simulink model "Quadcopter Plant Feedback"  (R2023a)
settings: Solver=VariableStepAuto  StartTime=0.0  StopTime=10.0  RelTol=1e-3
undefined symbols (not defined in the file): Ax, Ay, b, d, g, Ixx, Izz, Jr, m
settings Model: Creator=NADJICH  LastModifiedBy=NADJICH

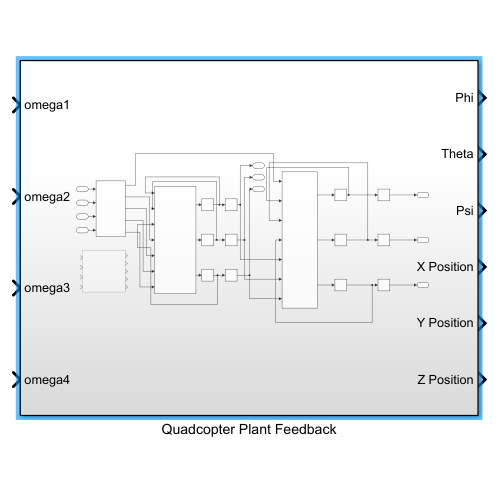
[thumbnail: Simulink's stored preview of the top-level diagram]
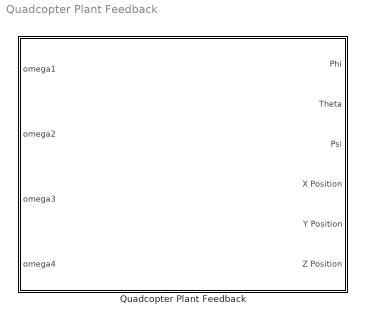
== system Quadcopter Plant Feedback ==
  Quadcopter Plant Feedback : Subsystem

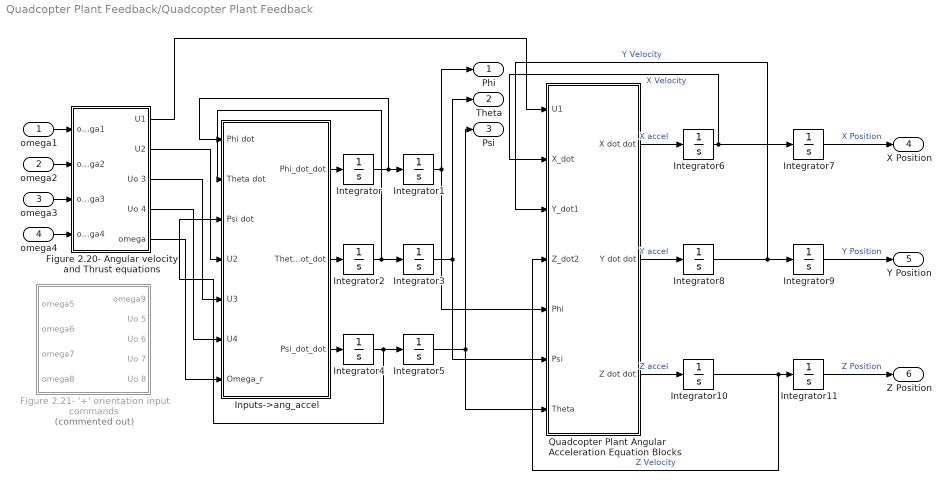
== system Quadcopter Plant Feedback/Quadcopter Plant Feedback ==
  omega1 : Inport
  omega2 : Inport  Port=2
  omega3 : Inport  Port=3
  omega4 : Inport  Port=4
  Figure 2.20- Angular velocity and Thrust equations : Subsystem
  Figure 2.21- '+' orientation input commands : Subsystem  Commented=on
  Inputs->ang_accel : Subsystem
  Integrator{,1..11} (12 alike) : Integrator
  Quadcopter Plant Angular Acceleration Equation Blocks : Subsystem
  Phi : Outport
  Theta : Outport  Port=2
  Psi : Outport  Port=3
  X Position : Outport  Port=4
  Y Position : Outport  Port=5
  Z Position : Outport  Port=6
  wires:
  omega1/1 -> Figure 2.20- Angular velocity and Thrust equations/1(omega1)
  omega2/1 -> Figure 2.20- Angular velocity and Thrust equations/2(omega2)
  omega3/1 -> Figure 2.20- Angular velocity and Thrust equations/3(omega3)
  omega4/1 -> Figure 2.20- Angular velocity and Thrust equations/4(omega4)
  Figure 2.20- Angular velocity and Thrust equations/5(omega) -> Inputs->ang_accel/7(Omega_r)
  Figure 2.20- Angular velocity and Thrust equations/2(U2) -> Inputs->ang_accel/4(U2)
  Figure 2.20- Angular velocity and Thrust equations/3(Uo 3) -> Inputs->ang_accel/5(U3)
  Figure 2.20- Angular velocity and Thrust equations/4(Uo 4) -> Inputs->ang_accel/6(U4)
  Inputs->ang_accel/1(Phi_dot_dot) -> Integrator/1
  Integrator/1 -> Integrator1/1, Inputs->ang_accel/1(Phi dot)
  Integrator2/1 -> Integrator3/1, Inputs->ang_accel/2(Theta dot)
  Integrator4/1 -> Integrator5/1, Inputs->ang_accel/3(Psi dot)
  Inputs->ang_accel/2(Theta_dot_dot) -> Integrator2/1
  Inputs->ang_accel/3(Psi_dot_dot) -> Integrator4/1
  Integrator1/1 -> Phi/1, Quadcopter Plant Angular Acceleration Equation Blocks/5(Phi)
  Integrator3/1 -> Theta/1, Quadcopter Plant Angular Acceleration Equation Blocks/6(Psi)
  Integrator5/1 -> Psi/1, Quadcopter Plant Angular Acceleration Equation Blocks/7(Theta)
  Figure 2.20- Angular velocity and Thrust equations/1(U1) -> Quadcopter Plant Angular Acceleration Equation Blocks/1(U1)
  Quadcopter Plant Angular Acceleration Equation Blocks/1(X dot dot) -> Integrator6/1  "X accel"
  Quadcopter Plant Angular Acceleration Equation Blocks/2(Y dot dot) -> Integrator8/1  "Y accel"
  Quadcopter Plant Angular Acceleration Equation Blocks/3(Z dot dot) -> Integrator10/1  "Z accel"
  Integrator6/1 -> Quadcopter Plant Angular Acceleration Equation Blocks/2(X_dot), Integrator7/1  "X Velocity"
  Integrator7/1 -> X Position/1  "X Position"
  Integrator8/1 -> Quadcopter Plant Angular Acceleration Equation Blocks/3(Y_dot1), Integrator9/1  "Y Velocity"
  Integrator9/1 -> Y Position/1  "Y Position"
  Integrator10/1 -> Integrator11/1, Quadcopter Plant Angular Acceleration Equation Blocks/4(Z_dot2)  "Z Velocity"
  Integrator11/1 -> Z Position/1  "Z Position"

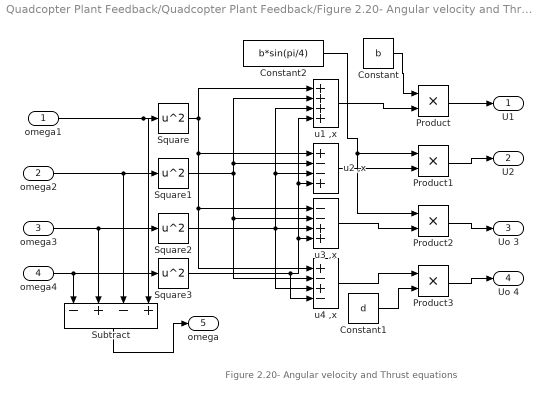
== system Quadcopter Plant Feedback/Quadcopter Plant Feedback/Figure 2.20- Angular velocity and Thrust equations ==
  note: Figure 2.20- Angular velocity and Thrust equations
  omega1 : Inport
  omega2 : Inport  Port=2
  omega3 : Inport  Port=3
  omega4 : Inport  Port=4
  Constant : Constant  Value=b
  Constant1 : Constant  Value=d
  Constant2 : Constant  Value=b*sin(pi/4)
  Product{,1..3} (4 alike) : Product
  Square{,1..3} (4 alike) : Math  Operator=square
  Subtract : Sum  Inputs=-+-+
  u1 ,x : Sum  Inputs=++++
  u2 ,x : Sum  Inputs=+--+
  u3 ,x : Sum  Inputs=--++
  u4 ,x : Sum  Inputs=+-+-
  U1 : Outport
  U2 : Outport  Port=2
  Uo 3 : Outport  Port=3
  Uo 4 : Outport  Port=4
  omega : Outport  Port=5
  wires:
  Constant/1 -> Product/1
  Product1/1 -> U2/1
  u4 ,x/1 -> Product3/1
  omega4/1 -> Square3/1, Subtract/1
  Square3/1 -> u4 ,x/4, u3 ,x/4, u2 ,x/4, u1 ,x/4
  omega1/1 -> Square/1, Subtract/4
  Product/1 -> U1/1
  Square1/1 -> u2 ,x/2, u1 ,x/2, u4 ,x/2, u3 ,x/2
  u3 ,x/1 -> Product2/2
  omega3/1 -> Subtract/2, Square2/1
  u1 ,x/1 -> Product/2
  Constant1/1 -> Product3/2
  Constant2/1 -> Product1/1, Product2/1
  omega2/1 -> Subtract/3, Square1/1
  Square/1 -> u4 ,x/1, u3 ,x/1, u2 ,x/1, u1 ,x/1
  Square2/1 -> u4 ,x/3, u3 ,x/3, u1 ,x/3, u2 ,x/3
  Product2/1 -> Uo 3/1
  Subtract/1 -> omega/1
  Product3/1 -> Uo 4/1
  u2 ,x/1 -> Product1/2

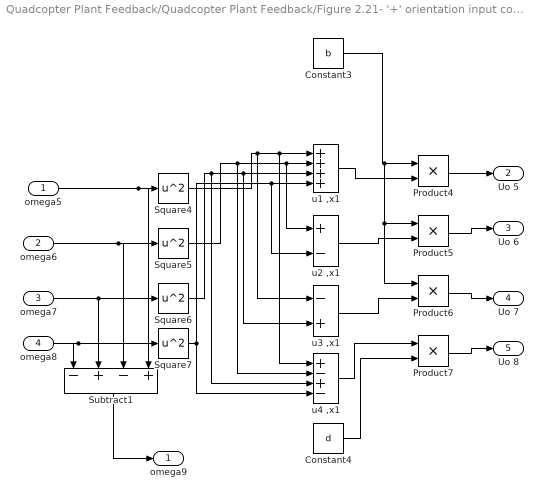
== system Quadcopter Plant Feedback/Quadcopter Plant Feedback/Figure 2.21- '+' orientation input commands ==
  omega5 : Inport
  omega6 : Inport  Port=2
  omega7 : Inport  Port=3
  omega8 : Inport  Port=4
  Constant3 : Constant  Value=b
  Constant4 : Constant  Value=d
  Product{4..7} (4 alike) : Product
  Square{4..7} (4 alike) : Math  Operator=square
  Subtract1 : Sum  Inputs=-+-+
  u1 ,x1 : Sum  Inputs=++++
  u2 ,x1 : Sum  Inputs=+-
  u3 ,x1 : Sum  Inputs=-+
  u4 ,x1 : Sum  Inputs=+-+-
  omega9 : Outport
  Uo 5 : Outport  Port=2
  Uo 6 : Outport  Port=3
  Uo 7 : Outport  Port=4
  Uo 8 : Outport  Port=5
  wires:
  Square5/1 -> u4 ,x1/2, u2 ,x1/1, u1 ,x1/2
  Constant3/1 -> Product6/1, Product5/1, Product4/1
  Square4/1 -> u3 ,x1/1, u4 ,x1/1, u1 ,x1/1
  Product7/1 -> Uo 8/1
  Constant4/1 -> Product7/2
  omega6/1 -> Square5/1, Subtract1/3
  Product5/1 -> Uo 6/1
  Square7/1 -> u2 ,x1/2, u1 ,x1/4, u4 ,x1/4
  Product4/1 -> Uo 5/1
  u1 ,x1/1 -> Product4/2
  Square6/1 -> u4 ,x1/3, u3 ,x1/2, u1 ,x1/3
  omega8/1 -> Square7/1, Subtract1/1
  u2 ,x1/1 -> Product5/2
  Subtract1/1 -> omega9/1
  omega7/1 -> Square6/1, Subtract1/2
  omega5/1 -> Subtract1/4, Square4/1
  u3 ,x1/1 -> Product6/2
  Product6/1 -> Uo 7/1
  u4 ,x1/1 -> Product7/1

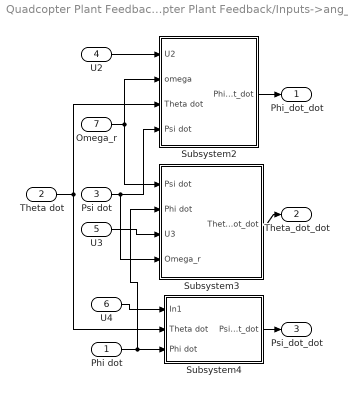
== system Quadcopter Plant Feedback/Quadcopter Plant Feedback/Inputs->ang_accel ==
  Phi dot : Inport
  Theta dot : Inport  Port=2
  Psi dot : Inport  Port=3
  U2 : Inport  Port=4
  U3 : Inport  Port=5
  U4 : Inport  Port=6
  Omega_r : Inport  Port=7
  Subsystem2 : Subsystem
  Subsystem3 : Subsystem
  Subsystem4 : Subsystem
  Phi_dot_dot : Outport
  Theta_dot_dot : Outport  Port=2
  Psi_dot_dot : Outport  Port=3
  wires:
  Subsystem4/1(Psi_dot_dot) -> Psi_dot_dot/1
  Psi dot/1 -> Subsystem3/4(Omega_r), Subsystem2/4(Psi dot)
  Phi dot/1 -> Subsystem3/2(Phi dot), Subsystem4/3(Phi dot)
  Omega_r/1 -> Subsystem3/1(Psi dot), Subsystem2/2(omega)
  Subsystem3/1(Theta_dot_dot) -> Theta_dot_dot/1
  Subsystem2/1(Phi_dot_dot) -> Phi_dot_dot/1
  Theta dot/1 -> Subsystem2/3(Theta dot), Subsystem4/2(Theta dot)
  U4/1 -> Subsystem4/1(In1)
  U2/1 -> Subsystem2/1(U2)
  U3/1 -> Subsystem3/3(U3)

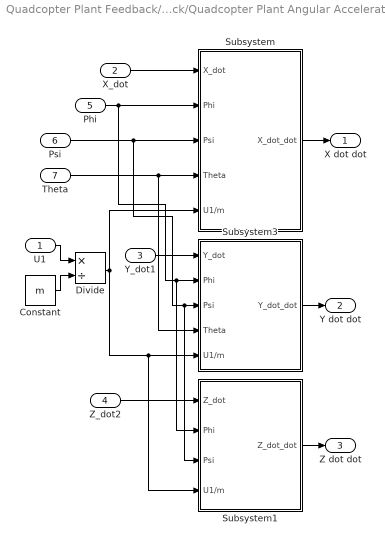
== system Quadcopter Plant Feedback/Quadcopter Plant Feedback/Quadcopter Plant Angular Acceleration Equation Blocks ==
  U1 : Inport
  X_dot : Inport  Port=2
  Y_dot1 : Inport  Port=3
  Z_dot2 : Inport  Port=4
  Phi : Inport  Port=5
  Psi : Inport  Port=6
  Theta : Inport  Port=7
  Constant : Constant  Value=m
  Divide : Product  Inputs=*/
  Subsystem : Subsystem
  Subsystem1 : Subsystem
  Subsystem3 : Subsystem
  X dot dot : Outport
  Y dot dot : Outport  Port=2
  Z dot dot : Outport  Port=3
  wires:
  Subsystem3/1(Y_dot_dot) -> Y dot dot/1
  U1/1 -> Divide/1
  Constant/1 -> Divide/2
  Subsystem/1(X_dot_dot) -> X dot dot/1
  Subsystem1/1(Z_dot_dot) -> Z dot dot/1
  X_dot/1 -> Subsystem/1(X_dot)
  Divide/1 -> Subsystem1/4(U1/m), Subsystem3/5(U1/m), Subsystem/5(U1/m)
  Y_dot1/1 -> Subsystem3/1(Y_dot)
  Phi/1 -> Subsystem1/2(Phi), Subsystem3/2(Phi), Subsystem/2(Phi)
  Theta/1 -> Subsystem3/4(Theta), Subsystem/4(Theta)
  Psi/1 -> Subsystem1/3(Psi), Subsystem3/3(Psi), Subsystem/3(Psi)
  Z_dot2/1 -> Subsystem1/1(Z_dot)

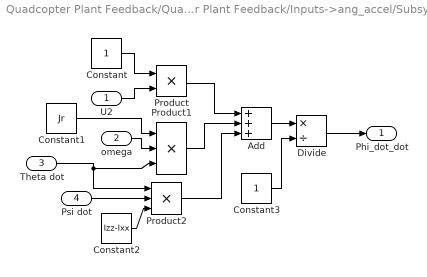
== system Quadcopter Plant Feedback/Quadcopter Plant Feedback/Inputs->ang_accel/Subsystem2 ==
  U2 : Inport
  omega : Inport  Port=2
  Theta dot : Inport  Port=3
  Psi dot : Inport  Port=4
  Add : Sum  Inputs=+++
  Constant : Constant
  Constant1 : Constant  Value=Jr
  Constant2 : Constant  Value=Izz-Ixx
  Constant3 : Constant
  Divide : Product  Inputs=*/
  Product : Product
  Product1 : Product  Inputs=3
  Product2 : Product  Inputs=3
  Phi_dot_dot : Outport
  wires:
  Add/1 -> Divide/1
  Divide/1 -> Phi_dot_dot/1
  Constant2/1 -> Product2/3
  Product2/1 -> Add/3
  U2/1 -> Product/2
  Product/1 -> Add/1
  Constant/1 -> Product/1
  Product1/1 -> Add/2
  Constant1/1 -> Product1/1
  Constant3/1 -> Divide/2
  omega/1 -> Product1/2
  Theta dot/1 -> Product2/1, Product1/3
  Psi dot/1 -> Product2/2

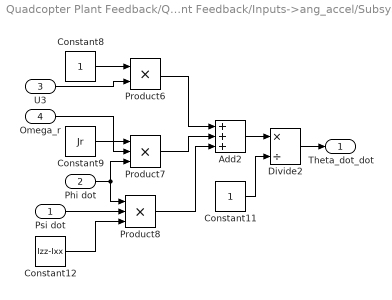
== system Quadcopter Plant Feedback/Quadcopter Plant Feedback/Inputs->ang_accel/Subsystem3 ==
  Psi dot : Inport
  Phi dot : Inport  Port=2
  U3 : Inport  Port=3
  Omega_r : Inport  Port=4
  Add2 : Sum  Inputs=+++
  Constant11 : Constant
  Constant12 : Constant  Value=Izz-Ixx
  Constant8 : Constant
  Constant9 : Constant  Value=Jr
  Divide2 : Product  Inputs=*/
  Product6 : Product
  Product7 : Product  Inputs=3
  Product8 : Product  Inputs=3
  Theta_dot_dot : Outport
  wires:
  Divide2/1 -> Theta_dot_dot/1
  Product7/1 -> Add2/2
  Add2/1 -> Divide2/1
  Constant9/1 -> Product7/1
  Product8/1 -> Add2/3
  Constant12/1 -> Product8/3
  Constant11/1 -> Divide2/2
  Product6/1 -> Add2/1
  Constant8/1 -> Product6/1
  Phi dot/1 -> Product7/3, Product8/1
  Psi dot/1 -> Product8/2
  Omega_r/1 -> Product7/2
  U3/1 -> Product6/2

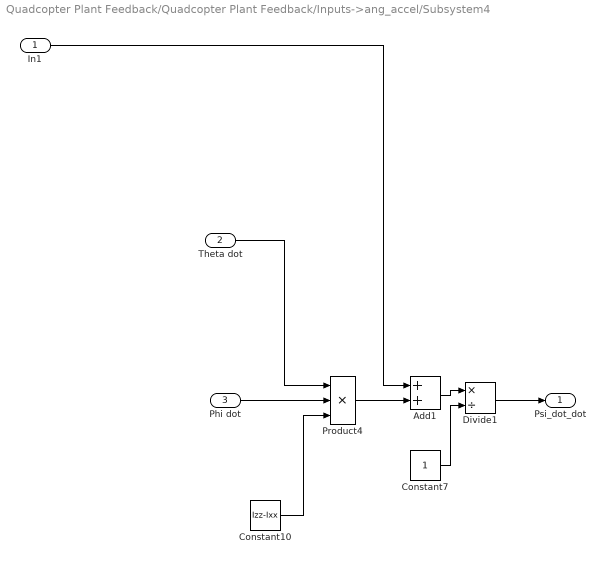
== system Quadcopter Plant Feedback/Quadcopter Plant Feedback/Inputs->ang_accel/Subsystem4 ==
  In1 : Inport
  Theta dot : Inport  Port=2
  Phi dot : Inport  Port=3
  Add1 : Sum
  Constant10 : Constant  Value=Izz-Ixx
  Constant7 : Constant
  Divide1 : Product  Inputs=*/
  Product4 : Product  Inputs=3
  Psi_dot_dot : Outport
  wires:
  Constant10/1 -> Product4/3
  Product4/1 -> Add1/2
  Divide1/1 -> Psi_dot_dot/1
  In1/1 -> Add1/1
  Constant7/1 -> Divide1/2
  Add1/1 -> Divide1/1
  Phi dot/1 -> Product4/2
  Theta dot/1 -> Product4/1

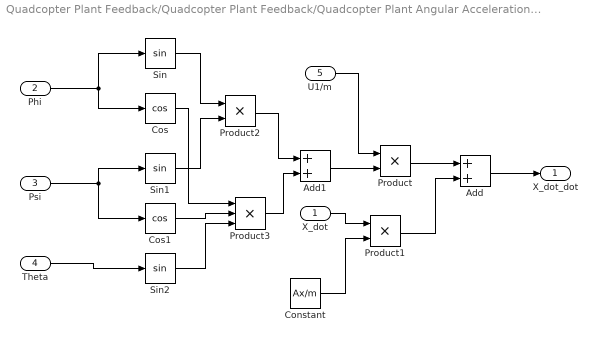
== system Quadcopter Plant Feedback/Quadcopter Plant Feedback/Quadcopter Plant Angular Acceleration Equation Blocks/Subsystem ==
  X_dot : Inport
  Phi : Inport  Port=2
  Psi : Inport  Port=3
  Theta : Inport  Port=4
  U1/m : Inport  Port=5
  Add : Sum
  Add1 : Sum
  Constant : Constant  Value=Ax/m
  Cos : Trigonometry  Operator=cos
  Cos1 : Trigonometry  Operator=cos
  Product : Product
  Product1 : Product
  Product2 : Product
  Product3 : Product  Inputs=3
  Sin : Trigonometry
  Sin1 : Trigonometry
  Sin2 : Trigonometry
  X_dot_dot : Outport
  wires:
  Phi/1 -> Sin/1, Cos/1
  Psi/1 -> Cos1/1, Sin1/1
  Theta/1 -> Sin2/1
  Sin1/1 -> Product2/2
  Sin/1 -> Product2/1
  Cos/1 -> Product3/1
  Cos1/1 -> Product3/2
  Sin2/1 -> Product3/3
  Product3/1 -> Add1/2
  Product2/1 -> Add1/1
  Add1/1 -> Product/2
  U1/m/1 -> Product/1
  X_dot/1 -> Product1/1
  Constant/1 -> Product1/2
  Product1/1 -> Add/2
  Product/1 -> Add/1
  Add/1 -> X_dot_dot/1

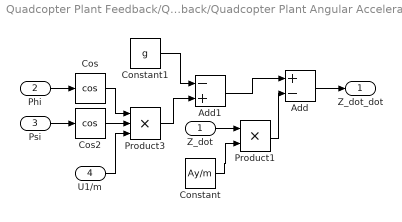
== system Quadcopter Plant Feedback/Quadcopter Plant Feedback/Quadcopter Plant Angular Acceleration Equation Blocks/Subsystem1 ==
  Z_dot : Inport
  Phi : Inport  Port=2
  Psi : Inport  Port=3
  U1/m : Inport  Port=4
  Add : Sum  Inputs=+-
  Add1 : Sum  Inputs=-+
  Constant : Constant  Value=Ay/m
  Constant1 : Constant  Value=g
  Cos : Trigonometry  Operator=cos
  Cos2 : Trigonometry  Operator=cos
  Product1 : Product
  Product3 : Product  Inputs=3
  Z_dot_dot : Outport
  wires:
  Phi/1 -> Cos/1
  Psi/1 -> Cos2/1
  Cos/1 -> Product3/1
  Product3/1 -> Add1/2
  Z_dot/1 -> Product1/1
  Constant/1 -> Product1/2
  Product1/1 -> Add/2
  Add/1 -> Z_dot_dot/1
  Constant1/1 -> Add1/1
  Cos2/1 -> Product3/2
  U1/m/1 -> Product3/3
  Add1/1 -> Add/1

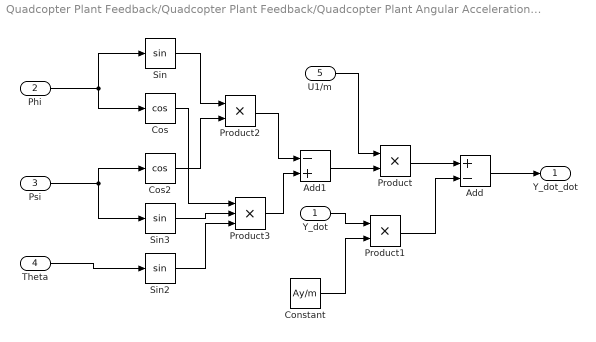
== system Quadcopter Plant Feedback/Quadcopter Plant Feedback/Quadcopter Plant Angular Acceleration Equation Blocks/Subsystem3 ==
  Y_dot : Inport
  Phi : Inport  Port=2
  Psi : Inport  Port=3
  Theta : Inport  Port=4
  U1/m : Inport  Port=5
  Add : Sum  Inputs=+-
  Add1 : Sum  Inputs=-+
  Constant : Constant  Value=Ay/m
  Cos : Trigonometry  Operator=cos
  Cos2 : Trigonometry  Operator=cos
  Product : Product
  Product1 : Product
  Product2 : Product
  Product3 : Product  Inputs=3
  Sin : Trigonometry
  Sin2 : Trigonometry
  Sin3 : Trigonometry
  Y_dot_dot : Outport
  wires:
  Add/1 -> Y_dot_dot/1
  Product/1 -> Add/1
  Product1/1 -> Add/2
  Constant/1 -> Product1/2
  Y_dot/1 -> Product1/1
  U1/m/1 -> Product/1
  Add1/1 -> Product/2
  Product2/1 -> Add1/1
  Product3/1 -> Add1/2
  Sin2/1 -> Product3/3
  Sin3/1 -> Product3/2
  Cos/1 -> Product3/1
  Sin/1 -> Product2/1
  Cos2/1 -> Product2/2
  Theta/1 -> Sin2/1
  Psi/1 -> Cos2/1, Sin3/1
  Phi/1 -> Cos/1, Sin/1
